simulink model "alp_sim"  (R2019a)
settings: Solver=VariableStepAuto  StartTime=0.0  StopTime=600  MaxStep=.01  RelTol=1e-3
libraries: simulink x2
settings Model: Creator=wifet  LastModifiedBy=wifet

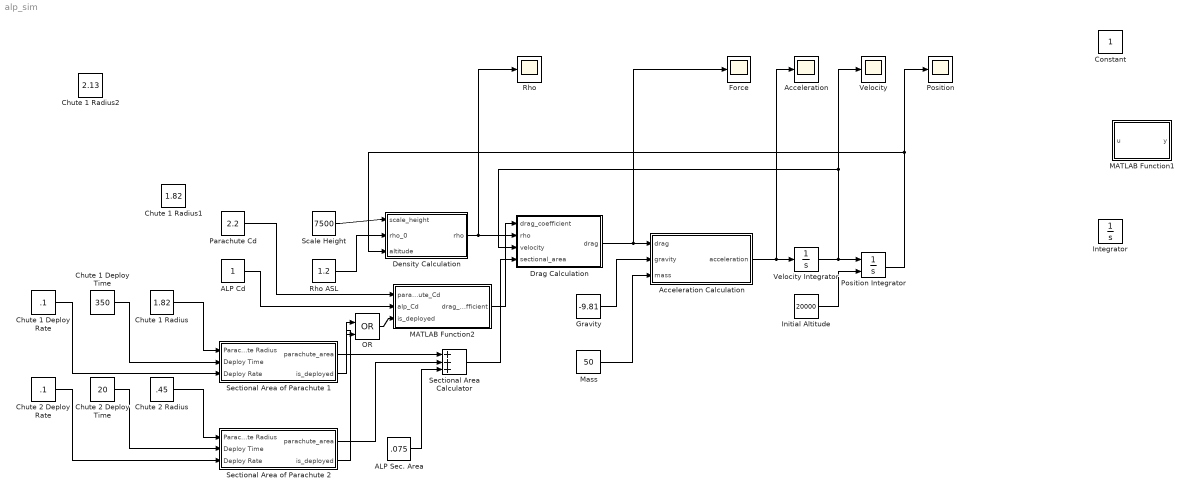
== system alp_sim ==
  ALP Cd : Constant
  ALP Sec. Area : Constant  Value=.075
  Acceleration : Scope
  Acceleration Calculation : MATLAB Function  TreatAsAtomicUnit=on
  Chute 1 Deploy Rate : Constant  Value=.1
  Chute 1 Deploy Time : Constant  Value=350
  Chute 1 Radius : Constant  Value=1.82
  Chute 1 Radius1 : Constant  Value=1.82
  Chute 1 Radius2 : Constant  Value=2.13
  Chute 2 Deploy Rate : Constant  Value=.1
  Chute 2 Deploy Time : Constant  Value=20
  Chute 2 Radius : Constant  Value=.45
  Constant : Constant
  Density Calculation : MATLAB Function  TreatAsAtomicUnit=on
  Drag Calculation : MATLAB Function  TreatAsAtomicUnit=on
  Force : Scope
  Gravity : Constant  Value=-9.81
  Initial Altitude : Constant  Value=20000
  Integrator : Integrator
  MATLAB Function1 : MATLAB Function  TreatAsAtomicUnit=on
  MATLAB Function2 : MATLAB Function  TreatAsAtomicUnit=on
  Mass : Constant  Value=50
  OR : Logic  Operator=OR  IconShape=distinctive  AllPortsSameDT=off  OutDataTypeStr=boolean
  Parachute Cd : Constant  Value=2.2
  Position : Scope
  Position Integrator : Integrator  InitialConditionSource=external
  Rho : Scope
  Rho ASL : Constant  Value=1.2
  Scale Height : Constant  Value=7500
  Sectional Area Calculator : Sum  Inputs=+++
  Sectional Area of Parachute 1 : Subsystem
  Sectional Area of Parachute 2 : Subsystem
  Velocity : Scope
  Velocity Integrator : Integrator
  wires:
  Drag Calculation/1(drag) -> Force/1, Acceleration Calculation/1(drag)
  Velocity Integrator/1 -> Velocity/1, Drag Calculation/3(velocity), Position Integrator/1
  Acceleration Calculation/1(acceleration) -> Acceleration/1, Velocity Integrator/1
  Density Calculation/1(rho) -> Rho/1, Drag Calculation/2(rho)
  Position Integrator/1 -> Position/1, Density Calculation/3(altitude)
  Scale Height/1 -> Density Calculation/1(scale_height)
  Rho ASL/1 -> Density Calculation/2(rho_0)
  Initial Altitude/1 -> Position Integrator/2
  Gravity/1 -> Acceleration Calculation/2(gravity)
  Mass/1 -> Acceleration Calculation/3(mass)
  Sectional Area Calculator/1 -> Drag Calculation/4(sectional_area)
  Sectional Area of Parachute 1/1(parachute_area) -> Sectional Area Calculator/1
  Sectional Area of Parachute 2/1(parachute_area) -> Sectional Area Calculator/2
  ALP Sec. Area/1 -> Sectional Area Calculator/3
  Sectional Area of Parachute 1/2(is_deployed) -> OR/1
  Sectional Area of Parachute 2/2(is_deployed) -> OR/2
  MATLAB Function2/1(drag_coefficient) -> Drag Calculation/1(drag_coefficient)
  OR/1 -> MATLAB Function2/3(is_deployed)
  Parachute Cd/1 -> MATLAB Function2/1(parachute_Cd)
  ALP Cd/1 -> MATLAB Function2/2(alp_Cd)
  Chute 1 Radius/1 -> Sectional Area of Parachute 1/1(Parachute Radius)
  Chute 1 Deploy Time/1 -> Sectional Area of Parachute 1/2(Deploy Time)
  Chute 1 Deploy Rate/1 -> Sectional Area of Parachute 1/3(Deploy Rate)
  Chute 2 Deploy Rate/1 -> Sectional Area of Parachute 2/3(Deploy Rate)
  Chute 2 Deploy Time/1 -> Sectional Area of Parachute 2/2(Deploy Time)
  Chute 2 Radius/1 -> Sectional Area of Parachute 2/1(Parachute Radius)

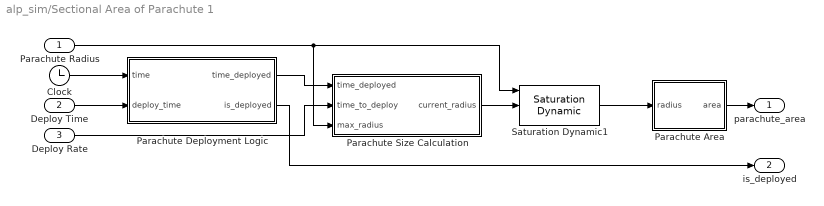
== system alp_sim/Sectional Area of Parachute 1 ==
  Parachute Radius : Inport
  Deploy Time : Inport  Port=2
  Deploy Rate : Inport  Port=3
  Clock : Clock
  Parachute Area : MATLAB Function  TreatAsAtomicUnit=on
  Parachute Deployment Logic : MATLAB Function  TreatAsAtomicUnit=on
  Parachute Size Calculation : MATLAB Function  TreatAsAtomicUnit=on
  Saturation Dynamic1 : simulink/Discontinuities/Saturation Dynamic  OutMin=[]  OutMax=[]  OutDataTypeStr=Inherit: Same as second input  OutDataType=fixdt(1, 16)  OutScaling=2^-10  DoSatur=off
  parachute_area : Outport
  is_deployed : Outport  Port=2
  wires:
  Deploy Time/1 -> Parachute Deployment Logic/2(deploy_time)
  Clock/1 -> Parachute Deployment Logic/1(time)
  Parachute Deployment Logic/1(time_deployed) -> Parachute Size Calculation/1(time_deployed)
  Deploy Rate/1 -> Parachute Size Calculation/2(time_to_deploy)
  Parachute Size Calculation/1(current_radius) -> Saturation Dynamic1/2
  Parachute Radius/1 -> Parachute Size Calculation/3(max_radius), Saturation Dynamic1/1
  Saturation Dynamic1/1 -> Parachute Area/1(radius)
  Parachute Area/1(area) -> parachute_area/1
  Parachute Deployment Logic/2(is_deployed) -> is_deployed/1

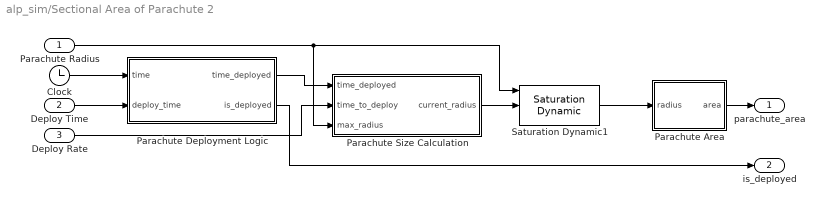
== system alp_sim/Sectional Area of Parachute 2 ==
  Parachute Radius : Inport
  Deploy Time : Inport  Port=2
  Deploy Rate : Inport  Port=3
  Clock : Clock
  Parachute Area : MATLAB Function  TreatAsAtomicUnit=on
  Parachute Deployment Logic : MATLAB Function  TreatAsAtomicUnit=on
  Parachute Size Calculation : MATLAB Function  TreatAsAtomicUnit=on
  Saturation Dynamic1 : simulink/Discontinuities/Saturation Dynamic  OutMin=[]  OutMax=[]  OutDataTypeStr=Inherit: Same as second input  OutDataType=fixdt(1, 16)  OutScaling=2^-10  DoSatur=off
  parachute_area : Outport
  is_deployed : Outport  Port=2
  wires:
  Deploy Time/1 -> Parachute Deployment Logic/2(deploy_time)
  Clock/1 -> Parachute Deployment Logic/1(time)
  Parachute Size Calculation/1(current_radius) -> Saturation Dynamic1/2
  Parachute Radius/1 -> Saturation Dynamic1/1, Parachute Size Calculation/3(max_radius)
  Saturation Dynamic1/1 -> Parachute Area/1(radius)
  Parachute Area/1(area) -> parachute_area/1
  Parachute Deployment Logic/2(is_deployed) -> is_deployed/1
  Deploy Rate/1 -> Parachute Size Calculation/2(time_to_deploy)
  Parachute Deployment Logic/1(time_deployed) -> Parachute Size Calculation/1(time_deployed)

== matlab function alp_sim/Density Calculation ==
  data: scale_height input; rho output; rho_0 input; altitude input
function rho = fcn(scale_height,rho_0,altitude)

rho = rho_0*2.71828^(-altitude/scale_height);

== matlab function alp_sim/Drag Calculation ==
  data: drag_coefficient input; drag output; rho input; velocity input; sectional_area input
function drag = fcn(drag_coefficient,rho,velocity,sectional_area)

drag = .5*drag_coefficient*rho*(velocity^2)*sectional_area;

== matlab function alp_sim/Acceleration Calculation ==
  data: drag input; acceleration output; gravity input; mass input
function acceleration = fcn(drag,gravity,mass)

acceleration = drag/mass+gravity;

== matlab function alp_sim/MATLAB Function1 ==
  data: u input; y output
function y = fcn(u)

y = u;

== matlab function alp_sim/Sectional Area of Parachute 1/Parachute Deployment Logic ==
  data: time input; time_deployed output; deploy_time input; is_deployed output
function [time_deployed,is_deployed]= fcn(time,deploy_time)
if time<deploy_time
    time_deployed=0;
    is_deployed=0;
else
    time_deployed = time-deploy_time;
    is_deployed=1;
end

== matlab function alp_sim/Sectional Area of Parachute 1/Parachute Size Calculation ==
  data: time_deployed input; current_radius output; time_to_deploy input; max_radius input
function current_radius = fcn(time_deployed,time_to_deploy,max_radius)

current_radius = (time_deployed*max_radius)/time_to_deploy;

== matlab function alp_sim/Sectional Area of Parachute 1/Parachute Area ==
  data: radius input; area output
function area = fcn(radius)

area = 3.14159265*radius^2;

== matlab function alp_sim/Sectional Area of Parachute 2/Parachute Area ==
  data: radius input; area output
function area = fcn(radius)

area = 3.14159265*radius^2;

== matlab function alp_sim/Sectional Area of Parachute 2/Parachute Deployment Logic ==
  data: time input; time_deployed output; deploy_time input; is_deployed output
function [time_deployed,is_deployed]= fcn(time,deploy_time)
if time<deploy_time
    time_deployed=0;
    is_deployed=0;
else
    time_deployed = time-deploy_time;
    is_deployed=1;
end

== matlab function alp_sim/Sectional Area of Parachute 2/Parachute Size Calculation ==
  data: time_deployed input; current_radius output; time_to_deploy input; max_radius input
function current_radius = fcn(time_deployed,time_to_deploy,max_radius)

current_radius = (time_deployed*max_radius)/time_to_deploy;

== matlab function alp_sim/MATLAB Function2 ==
  data: parachute_Cd input; drag_coefficient output; alp_Cd input; is_deployed input
function drag_coefficient= fcn(parachute_Cd,alp_Cd,is_deployed)
if is_deployed == 1
    drag_coefficient=parachute_Cd;
else
    drag_coefficient=alp_Cd;
end
